simulink model "Simplified_Model_test"  (R2014a)
settings: Solver=ode45  StartTime=0.0  StopTime=10  MinStep=0.01  RelTol=1e-3
libraries: simulink x6, rocket_vertical_flight_library x1, rocket_dynamic_data_library x1
settings Model: Creator=scorpii  LastModifiedBy=scorpii
settings SolverCC: InitialStep=0.01

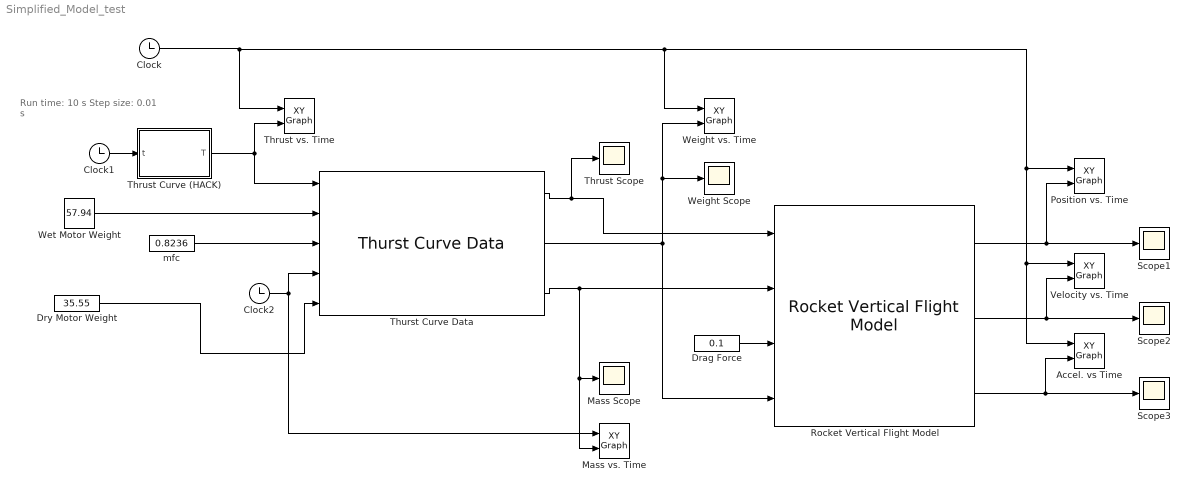
== system Simplified_Model_test ==
  note: Run time: 10 s
      | Step size: 0.01 s
  Accel. vs Time : simulink/Sinks/XY Graph  xmin=0  xmax=10  ymin=-1000  ymax=1000  st=-1
  Clock : Clock
  Clock1 : Clock
  Clock2 : Clock
  Drag Force : Constant  Value=0.1
  Dry Motor Weight : Constant  Value=35.55
  Mass Scope : Scope
      settings: SaveName=ScopeData5
  Mass vs. Time : simulink/Sinks/XY Graph  xmin=0  xmax=60  ymin=-10  ymax=100  st=-1
  Position vs. Time : simulink/Sinks/XY Graph  xmin=0  xmax=10  ymin=-20000  ymax=20000  st=-1
  Rocket Vertical Flight Model : rocket_vertical_flight_library/Rocket Vertical Flight Model
  Scope1 : Scope
  Scope2 : Scope
  Scope3 : Scope
      settings: SaveName=ScopeData2
  Thrust Curve (HACK) : MATLAB Function  TreatAsAtomicUnit=on
  "Thrust Scope " : Scope
      settings: SaveName=ScopeData3
  Thrust vs. Time : simulink/Sinks/XY Graph  xmin=0  xmax=10  ymin=-10  ymax=2500  st=-1
  Thurst Curve Data : rocket_dynamic_data_library/Thurst Curve Data
  Velocity vs. Time : simulink/Sinks/XY Graph  xmin=0  xmax=10  ymin=-1000  ymax=1000  st=-1
  Weight Scope : Scope
      settings: SaveName=ScopeData4
  Weight vs. Time : simulink/Sinks/XY Graph  xmin=0  xmax=10  ymin=-10  ymax=100  st=-1
  Wet Motor Weight : Constant  Value=57.94
  mfc : Constant  Value=0.8236
  wires:
  Rocket Vertical Flight Model/1 -> Position vs. Time/2, Scope1/1
  Rocket Vertical Flight Model/2 -> Velocity vs. Time/2, Scope2/1
  Rocket Vertical Flight Model/3 -> Accel. vs Time/2, Scope3/1
  mfc/1 -> Thurst Curve Data/3
  Thurst Curve Data/2 -> Weight Scope/1, Weight vs. Time/2, Rocket Vertical Flight Model/4
  Clock/1 -> Thrust vs. Time/1, Accel. vs Time/1, Velocity vs. Time/1, Position vs. Time/1, Weight vs. Time/1
  Wet Motor Weight/1 -> Thurst Curve Data/2
  Thurst Curve Data/3 -> Mass vs. Time/2, Mass Scope/1, Rocket Vertical Flight Model/2
  Drag Force/1 -> Rocket Vertical Flight Model/3
  Clock1/1 -> Thrust Curve (HACK)/1(t)
  Thrust Curve (HACK)/1(T) -> Thurst Curve Data/1, Thrust vs. Time/2
  Clock2/1 -> Mass vs. Time/1, Thurst Curve Data/4
  Thurst Curve Data/1 -> "Thrust Scope "/1, Rocket Vertical Flight Model/1
  Dry Motor Weight/1 -> Thurst Curve Data/5

== matlab function Simplified_Model_test/Thrust Curve (HACK) ==
  data: t input; T output
function T = thrust_hack(t)
    if t<0.08
    T=4000000*t^3-462933*t^2+41915*t+209.66
    elseif t<0.15935
    T=-4701*t+2748.7
    elseif t<0.21276 
    T=-1133.2*t+2223.6 
    elseif t<0.32775
    T=787.15*t+1850.2
    elseif t<0.57775
    T=-754.4*t+2339.9
    elseif t<0.72775
    T=-251*t+2070.7 
    elseif t<1.7277
    T=-70.147*t+1947.4
    elseif t<3.3777
    T=-31.421*t^2-9.1503*t+1930.8
    elseif t<3.9777
    T=3656.6*t^3-39167*t^2+137806*t-158018
    elseif t<4.5277
    T=-1051.8*t+4709.4
    else
    T=0
end
